simulink model "gm_uz_inverter_3phgm_vnl"  (R2021b)
settings: Solver=FixedStepDiscrete  StartTime=0.0  StopTime=0.6  FixedStep=Auto  RelTol=1e-3
InitFcn:
  | load('C:\Users\valen\Documents\repos\UZ\ultrazohm_sw\ip_cores\uz_inverter_3ph\sschdl\uz_inverter_3ph\stateSpaceParameters.mat');
undefined symbols (not defined in the file or in its folder): g1, g2, g3, g4, g5, g6, i_a, i_b, i_c, pslcontrol, stateSpaceParameters_1, ts
libraries: hdlmdlgenlib x20, simulink x4, hdlssclib x4
settings Model: Creator=LENOVO  LastModifiedBy=valen
settings SolverCC: AlgebraicLoopSolver=TrustRegion
settings DataIOCC: LimitDataPoints=on  SaveOutput=off  SaveTime=off
settings OptimizationCC: BlockReduction=off  ConditionallyExecuteInputs=off  DefaultParameterBehavior=Inlined  InheritOutputTypeSmallerThanSingle=on  LifeSpan=inf
settings DebuggingCC: AlgebraicLoopMsg=error  InheritedTsInSrcMsg=none  SingleTaskRateTransMsg=error  AllowSymbolicDim=off  StrictBusMsg=ErrorOnBusTreatedAsVector  SFUnexpectedBacktrackingDiag=warning  SFNoUnconditionalDefaultTransitionDiag=warning  SFExecutionAtInitializationDiag=none  SFMachineParentedDataDiag=warning  ArithmeticOperatorsInVariantConditions=warning
settings HardwareCC: ProdBitPerPointer=32  ProdBitPerSizeT=32  ProdBitPerPtrDiffT=32  ProdLargestAtomicFloat=None  ProdIntDivRoundTo=Undefined  ProdEndianess=Unspecified  ProdWordSize=32  ProdHWDeviceType=ASIC/FPGA->ASIC/FPGA  ProdEqTarget=off
settings SFSimCC: SimUseLocalCustomCode=off  CustomCodeUndefinedFunction=UseInterfaceOnly
settings RTWCC: RTWUseLocalCustomCode=off
settings CodeAppCC: StateflowObjectComments=on
settings GRTTargetCC: TargetLangStandard=C89/C90 (ANSI)
settings ConfigComp: CovScope=ReferencedModels  CovMetricSettings=dw  CovSaveCumulativeToWorkspaceVar=on  CovSaveSingleToWorkspaceVar=on  CovExternalEMLEnable=off  CovSFcnEnable=off

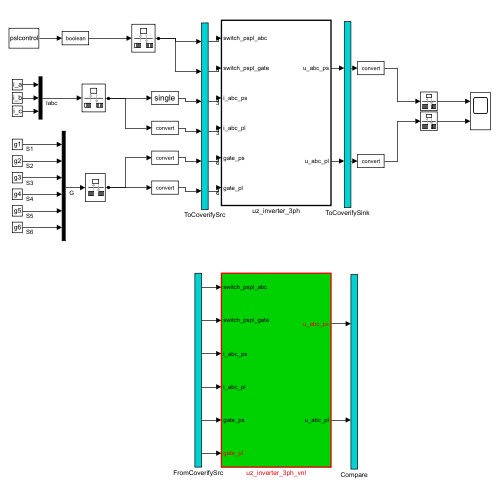
[thumbnail: Simulink's stored preview of the top-level diagram]
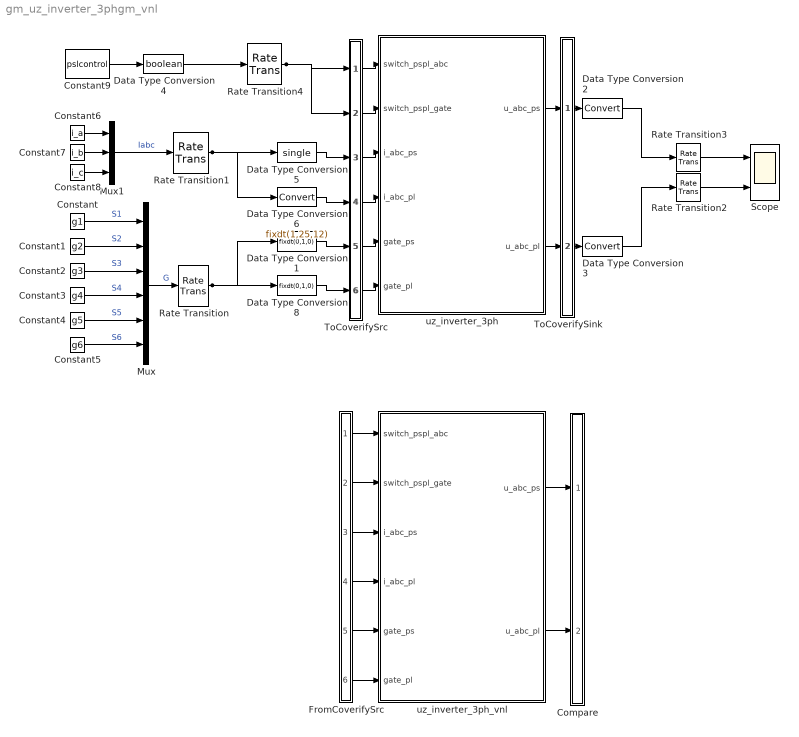
== system gm_uz_inverter_3phgm_vnl ==
  Compare : Subsystem
      mask Display: disp('')
  Constant : Constant  Value=g1  SampleTime=ts
  Constant1 : Constant  Value=g2  SampleTime=ts
  Constant2 : Constant  Value=g3  SampleTime=ts
  Constant3 : Constant  Value=g4  SampleTime=ts
  Constant4 : Constant  Value=g5  SampleTime=ts
  Constant5 : Constant  Value=g6  SampleTime=ts
  Constant6 : Constant  Value=i_a  SampleTime=ts
  Constant7 : Constant  Value=i_b  SampleTime=ts
  Constant8 : Constant  Value=i_c  SampleTime=ts
  Constant9 : Constant  Value=pslcontrol
  Data Type Conversion1 : DataTypeConversion  OutMin=0  OutMax=1  OutDataTypeStr=fixdt(0,1,0)  RndMeth=Nearest
  Data Type Conversion2 : DataTypeConversion
  Data Type Conversion3 : DataTypeConversion
  Data Type Conversion4 : DataTypeConversion  OutDataTypeStr=boolean
  Data Type Conversion5 : DataTypeConversion  OutDataTypeStr=single  RndMeth=Nearest
  Data Type Conversion6 : DataTypeConversion  OutDataTypeStr=fixdt(1,25,12)  RndMeth=Nearest
  Data Type Conversion8 : DataTypeConversion  OutMin=0  OutMax=1  OutDataTypeStr=fixdt(0,1,0)  RndMeth=Nearest
  FromCoverifySrc : Subsystem
      mask Display: disp('')
  Mux : Mux  Inputs=6
  Mux1 : Mux  Inputs=3
  Rate Transition{,1..4} (5 alike) : RateTransition  OutPortSampleTime=ts
  Scope : Scope  NumInputPorts=2
  ToCoverifySink : Subsystem
      mask Display: disp('')
  ToCoverifySrc : Subsystem
      mask Display: disp('')
  uz_inverter_3ph : Subsystem  TreatAsAtomicUnit=on
  uz_inverter_3ph_vnl : Subsystem  TreatAsAtomicUnit=on
  wires:
  Data Type Conversion3/1 -> Rate Transition2/1
  Data Type Conversion2/1 -> Rate Transition3/1
  Rate Transition3/1 -> Scope/1
  Rate Transition2/1 -> Scope/2
  Data Type Conversion4/1 -> Rate Transition4/1
  Constant9/1 -> Data Type Conversion4/1
  Constant2/1 -> Mux/3  "S3"
  Constant4/1 -> Mux/5  "S5"
  Constant5/1 -> Mux/6  "S6"
  Constant3/1 -> Mux/4  "S4"
  Mux1/1 -> Rate Transition1/1  "Iabc"
  Mux/1 -> Rate Transition/1  "G"
  Constant8/1 -> Mux1/3
  Constant6/1 -> Mux1/1
  Constant1/1 -> Mux/2  "S2"
  Constant7/1 -> Mux1/2
  Constant/1 -> Mux/1  "S1"
  Rate Transition1/1 -> Data Type Conversion5/1, Data Type Conversion6/1
  Rate Transition/1 -> Data Type Conversion8/1, Data Type Conversion1/1
  ToCoverifySrc/1(out1) -> uz_inverter_3ph/1(switch_pspl_abc)
  ToCoverifySrc/2(out2) -> uz_inverter_3ph/2(switch_pspl_gate)
  ToCoverifySrc/3(out3) -> uz_inverter_3ph/3(i_abc_ps)
  ToCoverifySrc/4(out4) -> uz_inverter_3ph/4(i_abc_pl)
  ToCoverifySrc/5(out5) -> uz_inverter_3ph/5(gate_ps)
  ToCoverifySrc/6(out6) -> uz_inverter_3ph/6(gate_pl)
  uz_inverter_3ph/1(u_abc_ps) -> ToCoverifySink/1(in1)
  uz_inverter_3ph/2(u_abc_pl) -> ToCoverifySink/2(in2)
  Rate Transition4/1 -> ToCoverifySrc/1(in1), ToCoverifySrc/2(in2)
  Data Type Conversion5/1 -> ToCoverifySrc/3(in3)
  Data Type Conversion6/1 -> ToCoverifySrc/4(in4)
  Data Type Conversion1/1 -> ToCoverifySrc/5(in5)
  Data Type Conversion8/1 -> ToCoverifySrc/6(in6)
  ToCoverifySink/1(out1) -> Data Type Conversion2/1
  ToCoverifySink/2(out2) -> Data Type Conversion3/1
  FromCoverifySrc/1(out1) -> uz_inverter_3ph_vnl/1(switch_pspl_abc)
  FromCoverifySrc/2(out2) -> uz_inverter_3ph_vnl/2(switch_pspl_gate)
  FromCoverifySrc/3(out3) -> uz_inverter_3ph_vnl/3(i_abc_ps)
  FromCoverifySrc/4(out4) -> uz_inverter_3ph_vnl/4(i_abc_pl)
  FromCoverifySrc/5(out5) -> uz_inverter_3ph_vnl/5(gate_ps)
  FromCoverifySrc/6(out6) -> uz_inverter_3ph_vnl/6(gate_pl)
  uz_inverter_3ph_vnl/1(u_abc_ps) -> Compare/1(in1)
  uz_inverter_3ph_vnl/2(u_abc_pl) -> Compare/2(in2)

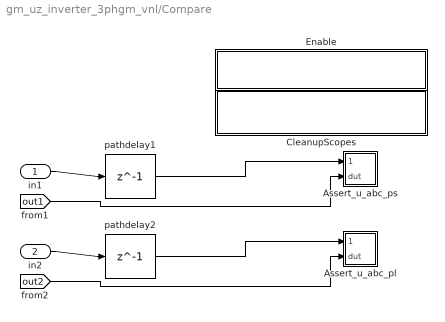
== system gm_uz_inverter_3phgm_vnl/Compare ==
  in1 : Inport
  in2 : Inport  Port=2
  Assert_u_abc_pl : Subsystem
  Assert_u_abc_ps : Subsystem  mask{ToleranceValue=0.001}
  CleanupScopes : Subsystem
      settings: OpenFcn=|
      | blkName = gcb; %self block
      | idx = regexp(blkName, '/CleanupScopes$', 'once');
      | blkParent = blkName(1:idx-1);
      | blks=find_system(blkParent, 'LookUnderMasks', 'all','blocktype', 'Scope');
      | for itr = 1:length(blks)
      | 	 hScopeCfg = get_param(blks{itr},'ScopeConfiguration');
      | 	 hScopeCfg.Visible = ~ hScopeCfg.Visible;
      | end
      | drawnow;
      mask Display: fprintf(message('hdlcoder:cosim:vnl_dblclick').getString());
  Enable : Subsystem
      settings: OpenFcn=|
      | blkName = gcb;
      | idx = regexp(blkName, '/Enable$', 'once');
      | blkParent = blkName(1:idx-1);
      | blks=find_system(blkParent, 'LookUnderMasks', 'all','blocktype', 'Assertion');
      | e = get_param(blks{1}, 'Enabled');
      | if strcmp(e, 'on'), f= 'off';, else, f = 'on';, end
      | for ii=1:length(blks), set_param(blks{ii}, 'Enabled', f);, end
      | set_param(gcb, 'MaskDisplay',['fprintf(message(''hdlcoder:cosim:vnl_dblclick_assertions'',','''',upper(e),'''',').getString())']);
      mask Display: fprintf(message('hdlcoder:cosim:vnl_dblclick_assertions','OFF').getString());
  pathdelay1 : Delay  DelayLength=1
  pathdelay2 : Delay  DelayLength=1
  wires:
  in1/1 -> pathdelay1/1
  pathdelay1/1 -> Assert_u_abc_ps/1(cosim)
  [out1] -> Assert_u_abc_ps/2(dut)
  in2/1 -> pathdelay2/1
  pathdelay2/1 -> Assert_u_abc_pl/1(cosim)
  [out2] -> Assert_u_abc_pl/2(dut)

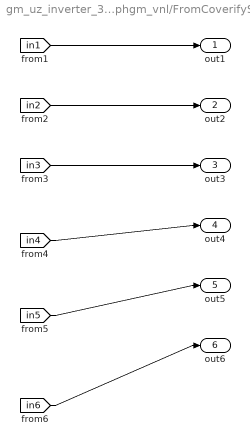
== system gm_uz_inverter_3phgm_vnl/FromCoverifySrc ==
  out1 : Outport
  out2 : Outport  Port=2
  out3 : Outport  Port=3
  out4 : Outport  Port=4
  out5 : Outport  Port=5
  out6 : Outport  Port=6
  wires:
  [in1] -> out1/1
  [in2] -> out2/1
  [in3] -> out3/1
  [in4] -> out4/1
  [in5] -> out5/1
  [in6] -> out6/1

== system gm_uz_inverter_3phgm_vnl/ToCoverifySink ==
  in1 : Inport
  in2 : Inport  Port=2
  out1 : Outport
  out2 : Outport  Port=2
  tag scope: out1=global, out2=global
  wires:
  in1/1 -> out1/1, [out1]
  in2/1 -> out2/1, [out2]

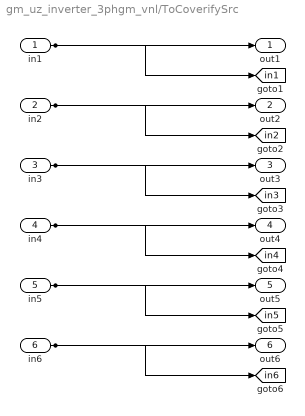
== system gm_uz_inverter_3phgm_vnl/ToCoverifySrc ==
  in1 : Inport
  in2 : Inport  Port=2
  in3 : Inport  Port=3
  in4 : Inport  Port=4
  in5 : Inport  Port=5
  in6 : Inport  Port=6
  out1 : Outport
  out2 : Outport  Port=2
  out3 : Outport  Port=3
  out4 : Outport  Port=4
  out5 : Outport  Port=5
  out6 : Outport  Port=6
  tag scope: in1=global, in2=global, in3=global, in4=global, in5=global, in6=global
  wires:
  in1/1 -> out1/1, [in1]
  in2/1 -> out2/1, [in2]
  in3/1 -> out3/1, [in3]
  in4/1 -> out4/1, [in4]
  in5/1 -> out5/1, [in5]
  in6/1 -> out6/1, [in6]

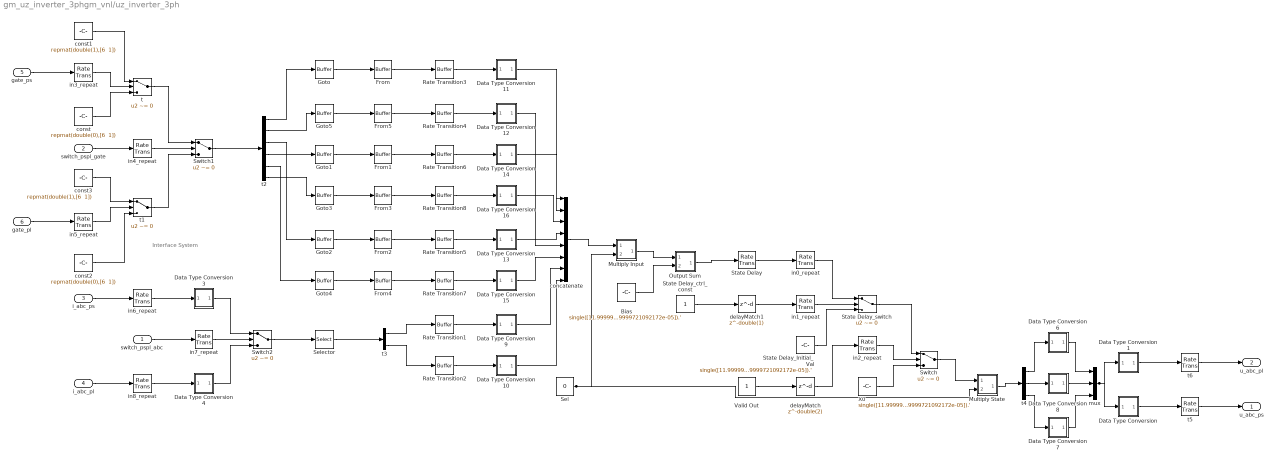
== system gm_uz_inverter_3phgm_vnl/uz_inverter_3ph ==
  note: Interface System
  switch_pspl_abc : Inport  OutDataTypeStr=boolean  PortDimensions=1  SampleTime=5e-07
  switch_pspl_gate : Inport  Port=2  OutDataTypeStr=boolean  PortDimensions=1  SampleTime=5e-07
  i_abc_ps : Inport  Port=3  OutDataTypeStr=single  PortDimensions=[3]  SampleTime=5e-07
  i_abc_pl : Inport  Port=4  OutDataTypeStr=fixdt(1, 25, 12)  PortDimensions=[3]  SampleTime=5e-07
  gate_ps : Inport  Port=5  OutDataTypeStr=fixdt(0, 1, 0)  PortDimensions=[6]  SampleTime=5e-07  LockScale=on
  gate_pl : Inport  Port=6  OutDataTypeStr=fixdt(0, 1, 0)  PortDimensions=[6]  SampleTime=5e-07
  Bias : Constant  Value=single([11.99999713897705 -11.99999713897705 0 -0.0002399999793851748 2.399999721092172e-05 -0.00012 1.2e-05 -2.6399995037285073e-11 0.00026399994385428727 0.00026399994385428727 1.2e-05 2.399999721092172e-05]).'  OutDataTypeStr=single  SampleTime=1e-08
  Data Type Conversion : Subsystem
      mask Display: disp('NFP\nconv');
  Data Type Conversion1 : Subsystem
      mask Display: disp('NFP\nconv');
  Data Type Conversion10 : Subsystem
      mask Display: disp('NFP\nconv');
  Data Type Conversion11 : Subsystem
      mask Display: disp('NFP\nconv');
  Data Type Conversion12 : Subsystem
      mask Display: disp('NFP\nconv');
  Data Type Conversion13 : Subsystem
      mask Display: disp('NFP\nconv');
  Data Type Conversion14 : Subsystem
      mask Display: disp('NFP\nconv');
  Data Type Conversion15 : Subsystem
      mask Display: disp('NFP\nconv');
  Data Type Conversion16 : Subsystem
      mask Display: disp('NFP\nconv');
  Data Type Conversion3 : Subsystem
      mask Display: disp('NFP\nconv');
  Data Type Conversion4 : Subsystem
      mask Display: disp('NFP\nconv');
  Data Type Conversion6 : Subsystem
      mask Display: disp('NFP\nconv');
  Data Type Conversion7 : Subsystem
      mask Display: disp('NFP\nconv');
  Data Type Conversion8 : Subsystem
      mask Display: disp('NFP\nconv');
  Data Type Conversion9 : Subsystem
      mask Display: disp('NFP\nconv');
  From{,1..5} (6 alike) : hdlmdlgenlib/Buffer
      settings: SourceProductBaseCode=SL
  Goto{,1..5} (6 alike) : hdlmdlgenlib/Buffer
      settings: SourceProductBaseCode=SL
  Multiply Input : Subsystem
      mask Display: disp('NFP\nSparseConstMultiply');
  Multiply State : Subsystem
      mask Display: disp('NFP\nSparseConstMultiply');
  Output Sum : Subsystem
      mask Display: disp('NFP\nadd');
  Rate Transition{1..8} (8 alike) : hdlmdlgenlib/Buffer
      settings: SourceProductBaseCode=SL
  Sel : Constant  Value=0  OutDataTypeStr=uint32  SampleTime=1e-08
  Selector : Selector  SampleTime=1e-08  IndexOptions=Index vector (dialog)  Indices=double([1 2])  OutputSizes=double(1)
  State Delay : RateTransition  OutPortSampleTimeOpt=Multiple of input port sample time  OutPortSampleTimeMultiple=50
  State Delay_Initial_Val : Constant  Value=single([11.99999713897705 -11.99999713897705 6.543061643369901e-16 -0.0002399999793851748 2.399999721092172e-05 -0.00012 1.2e-05 -2.6399995037285073e-11 0.00026399994385428727 0.00026399994385428727 1.2e-05 2.399999721092172e-05]).'  OutDataTypeStr=single  SampleTime=1e-08
  State Delay_ctrl_const : Constant  OutDataTypeStr=boolean  SampleTime=5e-07
  State Delay_switch : Switch  Criteria=u2 ~= 0  Threshold=double(0)  OutDataTypeStr=single  SampleTime=1e-08
  Switch : Switch  Criteria=u2 ~= 0  Threshold=double(0)  OutDataTypeStr=single  SampleTime=1e-08
  Switch1 : Switch  Criteria=u2 ~= 0  Threshold=double(0)  OutDataTypeStr=double  SampleTime=1e-08
  Switch2 : Switch  Criteria=u2 ~= 0  Threshold=double(0)  OutDataTypeStr=double  SampleTime=1e-08
  Valid Out : Constant  OutDataTypeStr=boolean  SampleTime=5e-07
  X0 : Constant  Value=single([11.99999713897705 -11.99999713897705 6.543061643369901e-16 -0.0002399999793851748 2.399999721092172e-05 -0.00012 1.2e-05 -2.6399995037285073e-11 0.00026399994385428727 0.00026399994385428727 1.2e-05 2.399999721092172e-05]).'  OutDataTypeStr=single  SampleTime=1e-08
  concatenate : Concatenate  NumInputs=8
  const : Constant  Value="repmat(double(0),[6  1])"  OutDataTypeStr=double  SampleTime=1e-08
  const1 : Constant  Value="repmat(double(1),[6  1])"  OutDataTypeStr=double  SampleTime=1e-08
  const2 : Constant  Value="repmat(double(0),[6  1])"  OutDataTypeStr=double  SampleTime=1e-08
  const3 : Constant  Value="repmat(double(1),[6  1])"  OutDataTypeStr=double  SampleTime=1e-08
  delayMatch : Delay  DelayLength=double(2)  InitialCondition=0  SampleTime=5e-07
  delayMatch1 : Delay  DelayLength=double(1)  InitialCondition=0  SampleTime=5e-07
  in0_repeat : RateTransition  Integrity=off  Deterministic=off  OutPortSampleTimeOpt=Multiple of input port sample time  OutPortSampleTimeMultiple=1/50
  in1_repeat : RateTransition  Integrity=off  Deterministic=off  OutPortSampleTimeOpt=Multiple of input port sample time  OutPortSampleTimeMultiple=1/50
  in2_repeat : RateTransition  Integrity=off  Deterministic=off  OutPortSampleTimeOpt=Multiple of input port sample time  OutPortSampleTimeMultiple=1/50
  in3_repeat : RateTransition  Integrity=off  Deterministic=off  OutPortSampleTimeOpt=Multiple of input port sample time  OutPortSampleTimeMultiple=1/50
  in4_repeat : RateTransition  Integrity=off  Deterministic=off  OutPortSampleTimeOpt=Multiple of input port sample time  OutPortSampleTimeMultiple=1/50
  in5_repeat : RateTransition  Integrity=off  Deterministic=off  OutPortSampleTimeOpt=Multiple of input port sample time  OutPortSampleTimeMultiple=1/50
  in6_repeat : RateTransition  Integrity=off  Deterministic=off  OutPortSampleTimeOpt=Multiple of input port sample time  OutPortSampleTimeMultiple=1/50
  in7_repeat : RateTransition  Integrity=off  Deterministic=off  OutPortSampleTimeOpt=Multiple of input port sample time  OutPortSampleTimeMultiple=1/50
  in8_repeat : RateTransition  Integrity=off  Deterministic=off  OutPortSampleTimeOpt=Multiple of input port sample time  OutPortSampleTimeMultiple=1/50
  mux : Mux  Inputs=3
  t : Switch  Criteria=u2 ~= 0  Threshold=double(0)  OutDataTypeStr=double  SampleTime=1e-08
  t1 : Switch  Criteria=u2 ~= 0  Threshold=double(0)  OutDataTypeStr=double  SampleTime=1e-08
  t2 : Demux  Outputs=6
  t3 : Demux  Outputs=2
  t4 : Demux  Outputs=3
  t5 : RateTransition  OutPortSampleTimeOpt=Multiple of input port sample time  OutPortSampleTimeMultiple=50
  t6 : RateTransition  OutPortSampleTimeOpt=Multiple of input port sample time  OutPortSampleTimeMultiple=50
  u_abc_ps : Outport  SampleTime=5e-07
  u_abc_pl : Outport  Port=2  OutDataTypeStr=fixdt(1,25,12)  SampleTime=5e-07
  wires:
  Data Type Conversion/1(Out1) -> t5/1
  Data Type Conversion6/1(Out1) -> mux/1
  Multiply State/1(Out1) -> t4/1
  Multiply Input/1(Out1) -> Output Sum/1(In1)
  Data Type Conversion9/1(Out1) -> concatenate/7
  Data Type Conversion4/1(Out1) -> Switch2/3
  Data Type Conversion3/1(Out1) -> Switch2/1
  Data Type Conversion10/1(Out1) -> concatenate/8
  Data Type Conversion11/1(Out1) -> concatenate/1
  Data Type Conversion16/1(Out1) -> concatenate/3
  Data Type Conversion15/1(Out1) -> concatenate/6
  Data Type Conversion14/1(Out1) -> concatenate/2
  Data Type Conversion13/1(Out1) -> concatenate/4
  Data Type Conversion12/1(Out1) -> concatenate/5
  Output Sum/1(Out1) -> State Delay/1
  Data Type Conversion7/1(Out1) -> mux/3
  Data Type Conversion8/1(Out1) -> mux/2
  Data Type Conversion1/1(Out1) -> t6/1
  t4/3 -> Data Type Conversion7/1(In1)
  t4/2 -> Data Type Conversion8/1(In1)
  t4/1 -> Data Type Conversion6/1(In1)
  t3/2 -> Rate Transition2/1
  t3/1 -> Rate Transition1/1
  t2/6 -> Goto3/1
  t2/5 -> Goto4/1
  t2/4 -> Goto1/1
  t2/3 -> Goto2/1
  t2/2 -> Goto5/1
  t2/1 -> Goto/1
  const3/1 -> t1/1
  const2/1 -> t1/3
  const1/1 -> t/1
  const/1 -> t/3
  mux/1 -> Data Type Conversion1/1(In1), Data Type Conversion/1(In1)
  Sel/1 -> Multiply Input/2(In2), Multiply State/2(In2)
  concatenate/1 -> Multiply Input/1(In1)
  Rate Transition1/1 -> Data Type Conversion9/1(In1)
  Selector/1 -> t3/1
  Switch2/1 -> Selector/1
  Rate Transition2/1 -> Data Type Conversion10/1(In1)
  Rate Transition3/1 -> Data Type Conversion11/1(In1)
  From/1 -> Rate Transition3/1
  Goto/1 -> From/1
  Switch1/1 -> t2/1
  t1/1 -> Switch1/3
  t/1 -> Switch1/1
  Goto3/1 -> From3/1
  From3/1 -> Rate Transition8/1
  Rate Transition8/1 -> Data Type Conversion16/1(In1)
  Goto4/1 -> From4/1
  From4/1 -> Rate Transition7/1
  Rate Transition7/1 -> Data Type Conversion15/1(In1)
  Goto1/1 -> From1/1
  From1/1 -> Rate Transition6/1
  Rate Transition6/1 -> Data Type Conversion14/1(In1)
  Goto2/1 -> From2/1
  From2/1 -> Rate Transition5/1
  Rate Transition5/1 -> Data Type Conversion13/1(In1)
  Goto5/1 -> From5/1
  From5/1 -> Rate Transition4/1
  Rate Transition4/1 -> Data Type Conversion12/1(In1)
  Bias/1 -> Output Sum/2(In2)
  Switch/1 -> Multiply State/1(In1)
  X0/1 -> Switch/3
  State Delay_switch/1 -> Switch/1
  State Delay_Initial_Val/1 -> State Delay_switch/3
  in8_repeat/1 -> Data Type Conversion4/1(In1)
  in7_repeat/1 -> Switch2/2
  in6_repeat/1 -> Data Type Conversion3/1(In1)
  in5_repeat/1 -> t1/2
  in4_repeat/1 -> Switch1/2
  in3_repeat/1 -> t/2
  in2_repeat/1 -> Switch/2
  in1_repeat/1 -> State Delay_switch/2
  in0_repeat/1 -> State Delay_switch/1
  State Delay_ctrl_const/1 -> delayMatch1/1
  Valid Out/1 -> delayMatch/1
  State Delay/1 -> in0_repeat/1
  t6/1 -> u_abc_pl/1
  t5/1 -> u_abc_ps/1
  delayMatch1/1 -> in1_repeat/1
  delayMatch/1 -> in2_repeat/1
  gate_pl/1 -> in5_repeat/1
  gate_ps/1 -> in3_repeat/1
  i_abc_pl/1 -> in8_repeat/1
  i_abc_ps/1 -> in6_repeat/1
  switch_pspl_gate/1 -> in4_repeat/1
  switch_pspl_abc/1 -> in7_repeat/1

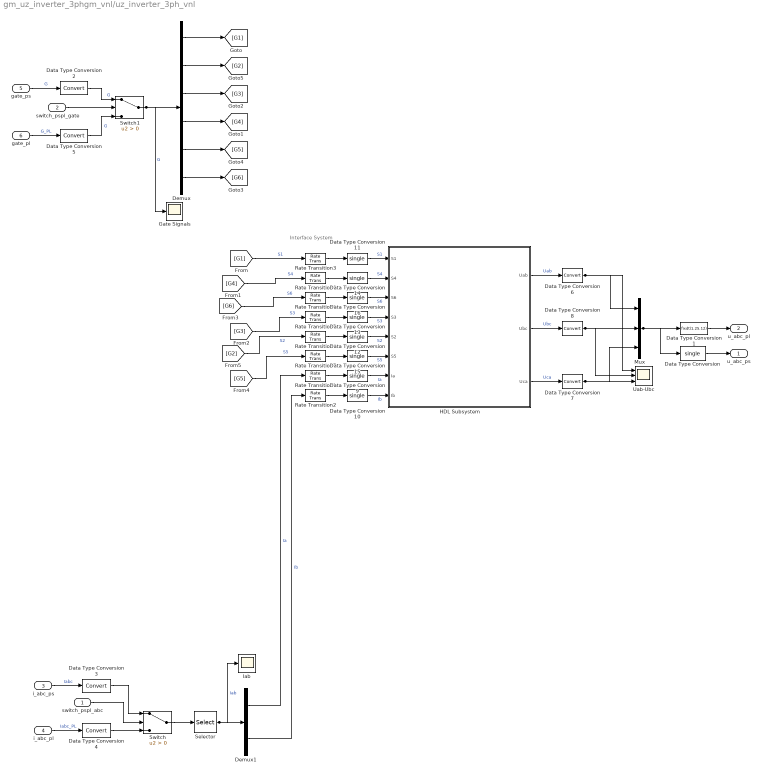
== system gm_uz_inverter_3phgm_vnl/uz_inverter_3ph_vnl ==
  note: Interface System
  switch_pspl_abc : Inport
  switch_pspl_gate : Inport  Port=2
  i_abc_ps : Inport  Port=3  OutDataTypeStr=single
  i_abc_pl : Inport  Port=4  OutDataTypeStr=fixdt(1,25,12)
  gate_ps : Inport  Port=5  OutDataTypeStr=fixdt(0,1,0)  LockScale=on
  gate_pl : Inport  Port=6  OutDataTypeStr=fixdt(0,1,0)
  Data Type Conversion{,9..16} (9 alike) : DataTypeConversion  OutDataTypeStr=single  RndMeth=Nearest
  Data Type Conversion1 : DataTypeConversion  OutDataTypeStr=fixdt(1,25,12)  RndMeth=Nearest
  Data Type Conversion{2..8} (7 alike) : DataTypeConversion  RndMeth=Nearest
  Demux : Demux  Outputs=6
  Demux1 : Demux  Outputs=2
  Gate Signals : Scope
  HDL Subsystem : Subsystem
  Iab : Scope
  Mux : Mux  Inputs=3
  Rate Transition{1..8} (8 alike) : RateTransition  OutPortSampleTime=5e-07
  Selector : Selector  InputPortWidth=3  IndexOptions=Index vector (dialog)  Indices=[1 2]  OutputSizes=1
  Switch : Switch  Criteria=u2 > Threshold
  Switch1 : Switch  Criteria=u2 > Threshold
  Uab-Ubc : Scope  NumInputPorts=3
  u_abc_ps : Outport
  u_abc_pl : Outport  Port=2  OutDataTypeStr=fixdt(1,25,12)
  wires:
  [G1] -> Rate Transition3/1  "S1"
  [G2] -> Rate Transition4/1  "S2"
  [G6] -> Rate Transition8/1  "S6"
  [G5] -> Rate Transition7/1  "S5"
  HDL Subsystem/1(Uab) -> Data Type Conversion6/1  "Uab"
  HDL Subsystem/3(Uca) -> Data Type Conversion7/1  "Uca"
  HDL Subsystem/2(Ubc) -> Data Type Conversion8/1  "Ubc"
  Demux1/1 -> Rate Transition1/1  "Ia"
  [G3] -> Rate Transition5/1  "S3"
  Demux1/2 -> Rate Transition2/1  "Ib"
  [G4] -> Rate Transition6/1  "S4"
  Rate Transition2/1 -> Data Type Conversion10/1
  Rate Transition4/1 -> Data Type Conversion12/1
  Rate Transition1/1 -> Data Type Conversion9/1
  Rate Transition5/1 -> Data Type Conversion13/1
  Rate Transition8/1 -> Data Type Conversion16/1
  Data Type Conversion11/1 -> HDL Subsystem/1(S1)  "S1"
  Data Type Conversion14/1 -> HDL Subsystem/2(S4)  "S4"
  Data Type Conversion16/1 -> HDL Subsystem/3(S6)  "S6"
  Rate Transition3/1 -> Data Type Conversion11/1
  Data Type Conversion15/1 -> HDL Subsystem/6(S5)  "S5"
  Data Type Conversion12/1 -> HDL Subsystem/5(S2)  "S2"
  Data Type Conversion13/1 -> HDL Subsystem/4(S3)  "S3"
  i_abc_ps/1 -> Data Type Conversion3/1  "Iabc"
  Data Type Conversion9/1 -> HDL Subsystem/7(Ia)  "Ia"
  switch_pspl_abc/1 -> Switch/2
  Selector/1 -> Iab/1, Demux1/1  "Iab"
  Rate Transition6/1 -> Data Type Conversion14/1
  Demux/3 -> [G3]
  Data Type Conversion3/1 -> Switch/1
  Demux/1 -> [G1]
  Data Type Conversion4/1 -> Switch/3
  gate_ps/1 -> Data Type Conversion2/1  "G"
  Rate Transition7/1 -> Data Type Conversion15/1
  Data Type Conversion10/1 -> HDL Subsystem/8(Ib)  "Ib"
  switch_pspl_gate/1 -> Switch1/2
  Demux/6 -> [G6]
  gate_pl/1 -> Data Type Conversion5/1  "G_PL"
  Demux/4 -> [G4]
  Data Type Conversion1/1 -> u_abc_pl/1
  Mux/1 -> Data Type Conversion1/1, Data Type Conversion/1
  Data Type Conversion/1 -> u_abc_ps/1
  Data Type Conversion5/1 -> Switch1/3  "G"
  Demux/5 -> [G5]
  Data Type Conversion8/1 -> Uab-Ubc/2, Mux/2
  i_abc_pl/1 -> Data Type Conversion4/1  "Iabc_PL"
  Data Type Conversion7/1 -> Mux/3, Uab-Ubc/3
  Switch/1 -> Selector/1
  Data Type Conversion6/1 -> Uab-Ubc/1, Mux/1
  Switch1/1 -> Gate Signals/1, Demux/1  "G"
  Data Type Conversion2/1 -> Switch1/1  "G"
  Demux/2 -> [G2]

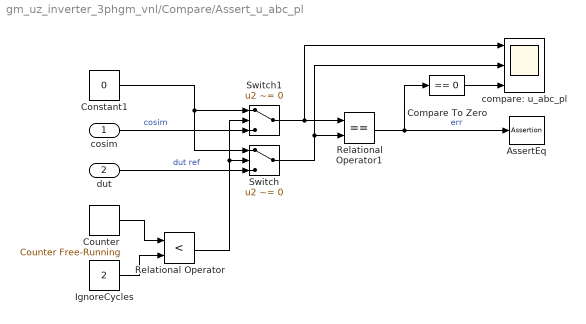
== system gm_uz_inverter_3phgm_vnl/Compare/Assert_u_abc_pl ==
  cosim : Inport
  dut : Inport  Port=2
  AssertEq : Assertion  StopWhenAssertionFail=off
  Compare To Zero : simulink/Logic and Bit Operations/Compare To Zero  relop===  OutDataTypeStr=boolean
  Constant1 : Constant  Value=0  OutDataTypeStr=Inherit: Inherit via back propagation  SampleTime=-1
  Counter : simulink/Sources/Counter Free-Running  NumBits=32  tsamp=-1
  IgnoreCycles : Constant  Value=2  OutDataTypeStr=Inherit: Inherit via back propagation  SampleTime=-1
  Relational Operator : RelationalOperator  Operator=<  OutDataTypeStr=boolean  RndMeth=Nearest
  Relational Operator1 : RelationalOperator  Operator===  OutDataTypeStr=boolean  RndMeth=Nearest
  Switch : Switch  Criteria=u2 ~= 0
  Switch1 : Switch  Criteria=u2 ~= 0
  compare: u_abc_pl : Scope  NumInputPorts=3
  wires:
  Compare To Zero/1 -> compare: u_abc_pl/3
  Relational Operator1/1 -> Compare To Zero/1, AssertEq/1  "err"
  Switch1/1 -> compare: u_abc_pl/1, Relational Operator1/1
  Switch/1 -> compare: u_abc_pl/2, Relational Operator1/2
  Constant1/1 -> Switch/1, Switch1/1
  Relational Operator/1 -> Switch/2, Switch1/2
  cosim/1 -> Switch1/3  "cosim"
  dut/1 -> Switch/3  "dut ref"
  Counter/1 -> Relational Operator/1
  IgnoreCycles/1 -> Relational Operator/2

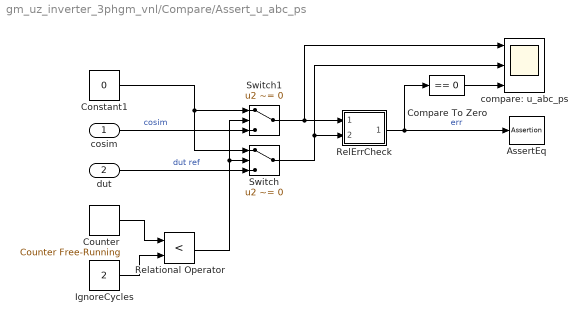
== system gm_uz_inverter_3phgm_vnl/Compare/Assert_u_abc_ps ==
  cosim : Inport
  dut : Inport  Port=2
  AssertEq : Assertion  StopWhenAssertionFail=off
  Compare To Zero : simulink/Logic and Bit Operations/Compare To Zero  relop===  OutDataTypeStr=boolean
  Constant1 : Constant  Value=0  OutDataTypeStr=Inherit: Inherit via back propagation  SampleTime=-1
  Counter : simulink/Sources/Counter Free-Running  NumBits=32  tsamp=-1
  IgnoreCycles : Constant  Value=2  OutDataTypeStr=Inherit: Inherit via back propagation  SampleTime=-1
  RelErrCheck : Subsystem
  Relational Operator : RelationalOperator  Operator=<  OutDataTypeStr=boolean  RndMeth=Nearest
  Switch : Switch  Criteria=u2 ~= 0
  Switch1 : Switch  Criteria=u2 ~= 0
  compare: u_abc_ps : Scope  NumInputPorts=3
  wires:
  IgnoreCycles/1 -> Relational Operator/2
  Counter/1 -> Relational Operator/1
  dut/1 -> Switch/3  "dut ref"
  cosim/1 -> Switch1/3  "cosim"
  Relational Operator/1 -> Switch1/2, Switch/2
  Constant1/1 -> Switch1/1, Switch/1
  Switch/1 -> compare: u_abc_ps/2, RelErrCheck/2(In2)
  Switch1/1 -> compare: u_abc_ps/1, RelErrCheck/1(In1)
  RelErrCheck/1(Out1) -> AssertEq/1, Compare To Zero/1  "err"
  Compare To Zero/1 -> compare: u_abc_ps/3

== system gm_uz_inverter_3phgm_vnl/Compare/CleanupScopes ==

== system gm_uz_inverter_3phgm_vnl/Compare/Enable ==

== system gm_uz_inverter_3phgm_vnl/uz_inverter_3ph/Data Type Conversion ==
  In1 : Inport
  Data Type Conversion : DataTypeConversion  OutDataTypeStr=single  RndMeth=Nearest  SampleTime=1e-08
  Data Type Conversion_pd1 : Delay  DelayLength=3
  Out1 : Outport
  wires:
  Data Type Conversion_pd1/1 -> Out1/1
  Data Type Conversion/1 -> Data Type Conversion_pd1/1
  In1/1 -> Data Type Conversion/1

== system gm_uz_inverter_3phgm_vnl/uz_inverter_3ph/Data Type Conversion1 ==
  In1 : Inport
  Data Type Conversion1 : DataTypeConversion  OutDataTypeStr=fixdt(1, 25, 12)  RndMeth=Nearest  SampleTime=1e-08
  Data Type Conversion1_pd1 : Delay  DelayLength=3
  Out1 : Outport
  wires:
  Data Type Conversion1_pd1/1 -> Out1/1
  Data Type Conversion1/1 -> Data Type Conversion1_pd1/1
  In1/1 -> Data Type Conversion1/1

== system gm_uz_inverter_3phgm_vnl/uz_inverter_3ph/Data Type Conversion10 ==
  In1 : Inport
  Data Type Conversion10 : DataTypeConversion  OutDataTypeStr=single  RndMeth=Nearest  SampleTime=1e-08
  Data Type Conversion10_pd1 : Delay  DelayLength=3
  Out1 : Outport
  wires:
  Data Type Conversion10_pd1/1 -> Out1/1
  Data Type Conversion10/1 -> Data Type Conversion10_pd1/1
  In1/1 -> Data Type Conversion10/1

== system gm_uz_inverter_3phgm_vnl/uz_inverter_3ph/Data Type Conversion11 ==
  In1 : Inport
  Data Type Conversion11 : DataTypeConversion  OutDataTypeStr=single  RndMeth=Nearest  SampleTime=1e-08
  Data Type Conversion11_pd1 : Delay  DelayLength=3
  Out1 : Outport
  wires:
  Data Type Conversion11_pd1/1 -> Out1/1
  Data Type Conversion11/1 -> Data Type Conversion11_pd1/1
  In1/1 -> Data Type Conversion11/1

== system gm_uz_inverter_3phgm_vnl/uz_inverter_3ph/Data Type Conversion12 ==
  In1 : Inport
  Data Type Conversion12 : DataTypeConversion  OutDataTypeStr=single  RndMeth=Nearest  SampleTime=1e-08
  Data Type Conversion12_pd1 : Delay  DelayLength=3
  Out1 : Outport
  wires:
  Data Type Conversion12_pd1/1 -> Out1/1
  Data Type Conversion12/1 -> Data Type Conversion12_pd1/1
  In1/1 -> Data Type Conversion12/1

== system gm_uz_inverter_3phgm_vnl/uz_inverter_3ph/Data Type Conversion13 ==
  In1 : Inport
  Data Type Conversion13 : DataTypeConversion  OutDataTypeStr=single  RndMeth=Nearest  SampleTime=1e-08
  Data Type Conversion13_pd1 : Delay  DelayLength=3
  Out1 : Outport
  wires:
  Data Type Conversion13_pd1/1 -> Out1/1
  Data Type Conversion13/1 -> Data Type Conversion13_pd1/1
  In1/1 -> Data Type Conversion13/1

== system gm_uz_inverter_3phgm_vnl/uz_inverter_3ph/Data Type Conversion14 ==
  In1 : Inport
  Data Type Conversion14 : DataTypeConversion  OutDataTypeStr=single  RndMeth=Nearest  SampleTime=1e-08
  Data Type Conversion14_pd1 : Delay  DelayLength=3
  Out1 : Outport
  wires:
  Data Type Conversion14_pd1/1 -> Out1/1
  Data Type Conversion14/1 -> Data Type Conversion14_pd1/1
  In1/1 -> Data Type Conversion14/1

== system gm_uz_inverter_3phgm_vnl/uz_inverter_3ph/Data Type Conversion15 ==
  In1 : Inport
  Data Type Conversion15 : DataTypeConversion  OutDataTypeStr=single  RndMeth=Nearest  SampleTime=1e-08
  Data Type Conversion15_pd1 : Delay  DelayLength=3
  Out1 : Outport
  wires:
  Data Type Conversion15_pd1/1 -> Out1/1
  Data Type Conversion15/1 -> Data Type Conversion15_pd1/1
  In1/1 -> Data Type Conversion15/1

== system gm_uz_inverter_3phgm_vnl/uz_inverter_3ph/Data Type Conversion16 ==
  In1 : Inport
  Data Type Conversion16 : DataTypeConversion  OutDataTypeStr=single  RndMeth=Nearest  SampleTime=1e-08
  Data Type Conversion16_pd1 : Delay  DelayLength=3
  Out1 : Outport
  wires:
  Data Type Conversion16_pd1/1 -> Out1/1
  Data Type Conversion16/1 -> Data Type Conversion16_pd1/1
  In1/1 -> Data Type Conversion16/1

== system gm_uz_inverter_3phgm_vnl/uz_inverter_3ph/Data Type Conversion3 ==
  In1 : Inport
  Data Type Conversion3 : DataTypeConversion  OutDataTypeStr=double  RndMeth=Nearest  SampleTime=1e-08
  Data Type Conversion3_pd1 : Delay  DelayLength=3
  Out1 : Outport
  wires:
  Data Type Conversion3_pd1/1 -> Out1/1
  Data Type Conversion3/1 -> Data Type Conversion3_pd1/1
  In1/1 -> Data Type Conversion3/1

== system gm_uz_inverter_3phgm_vnl/uz_inverter_3ph/Data Type Conversion4 ==
  In1 : Inport
  Data Type Conversion4 : DataTypeConversion  OutDataTypeStr=double  RndMeth=Nearest  SampleTime=1e-08
  Data Type Conversion4_pd1 : Delay  DelayLength=3
  Out1 : Outport
  wires:
  Data Type Conversion4_pd1/1 -> Out1/1
  Data Type Conversion4/1 -> Data Type Conversion4_pd1/1
  In1/1 -> Data Type Conversion4/1

== system gm_uz_inverter_3phgm_vnl/uz_inverter_3ph/Data Type Conversion6 ==
  In1 : Inport
  Data Type Conversion6 : DataTypeConversion  OutDataTypeStr=double  RndMeth=Nearest  SampleTime=1e-08
  Data Type Conversion6_pd1 : Delay  DelayLength=3
  Out1 : Outport
  wires:
  Data Type Conversion6_pd1/1 -> Out1/1
  Data Type Conversion6/1 -> Data Type Conversion6_pd1/1
  In1/1 -> Data Type Conversion6/1

== system gm_uz_inverter_3phgm_vnl/uz_inverter_3ph/Data Type Conversion7 ==
  In1 : Inport
  Data Type Conversion7 : DataTypeConversion  OutDataTypeStr=double  RndMeth=Nearest  SampleTime=1e-08
  Data Type Conversion7_pd1 : Delay  DelayLength=3
  Out1 : Outport
  wires:
  Data Type Conversion7_pd1/1 -> Out1/1
  Data Type Conversion7/1 -> Data Type Conversion7_pd1/1
  In1/1 -> Data Type Conversion7/1

== system gm_uz_inverter_3phgm_vnl/uz_inverter_3ph/Data Type Conversion8 ==
  In1 : Inport
  Data Type Conversion8 : DataTypeConversion  OutDataTypeStr=double  RndMeth=Nearest  SampleTime=1e-08
  Data Type Conversion8_pd1 : Delay  DelayLength=3
  Out1 : Outport
  wires:
  Data Type Conversion8_pd1/1 -> Out1/1
  Data Type Conversion8/1 -> Data Type Conversion8_pd1/1
  In1/1 -> Data Type Conversion8/1

== system gm_uz_inverter_3phgm_vnl/uz_inverter_3ph/Data Type Conversion9 ==
  In1 : Inport
  Data Type Conversion9 : DataTypeConversion  OutDataTypeStr=single  RndMeth=Nearest  SampleTime=1e-08
  Data Type Conversion9_pd1 : Delay  DelayLength=3
  Out1 : Outport
  wires:
  Data Type Conversion9_pd1/1 -> Out1/1
  Data Type Conversion9/1 -> Data Type Conversion9_pd1/1
  In1/1 -> Data Type Conversion9/1

== system gm_uz_inverter_3phgm_vnl/uz_inverter_3ph/Multiply Input ==
  In1 : Inport
  In2 : Inport  Port=2
  Multiply Input : hdlssclib/NFPSparseConstMultiply  constMatrix="reshape(single([0 0 0 0 0 0 0 0 0 0 0 0 0 0 0 0 0 0 0 0 0 0 0 0 0 0 0 0 0 0 0 0 0 0 0 0 0 0 0 0 0 0 0 0 0 0 0 0 0 0 0 0 0 0 0 0 0 0 0 0 0 0 0 0 0 0 0 0 0 0 0 0 -0.009999997913837433 0 45454.5469 9.999997985232767e-08 -9.999998162868451e-09 0.4545454680919647 -0.04545454680919647 0 0 0.9999997615814209 0.04545454680919647 0 0 -0.009999997913837433 45454.5469 0 0 0.4545454680919647 -0.04545454680919647 9.999997985232767e-08 -0.9999997615814209 0 0.04545454680919647 9.999998162868451e-09]).', [12   8])"
      settings: SourceProductBaseCode=SL
  Multiply Input_pd1 : Delay  DelayLength=12
  Out1 : Outport
  wires:
  Multiply Input_pd1/1 -> Out1/1
  Multiply Input/1 -> Multiply Input_pd1/1
  In2/1 -> Multiply Input/2
  In1/1 -> Multiply Input/1

== system gm_uz_inverter_3phgm_vnl/uz_inverter_3ph/Multiply State ==
  In1 : Inport
  In2 : Inport  Port=2
  Multiply State : hdlssclib/NFPSparseConstMultiply  constMatrix="reshape(single([1 0 -1 0 1 0 0 0 0 0 0 0 0 0 0 0 0 0 0 0 0 0 0 0 0 0 0 0 0 0 0 0 0 0 0 0]).', [3  12])"
      settings: SourceProductBaseCode=SL
  Multiply State_pd1 : Delay  DelayLength=6
  Out1 : Outport
  wires:
  Multiply State_pd1/1 -> Out1/1
  Multiply State/1 -> Multiply State_pd1/1
  In2/1 -> Multiply State/2
  In1/1 -> Multiply State/1

== system gm_uz_inverter_3phgm_vnl/uz_inverter_3ph/Output Sum ==
  In1 : Inport
  In2 : Inport  Port=2
  Output Sum : Sum  OutDataTypeStr=single  SampleTime=1e-08
  Output Sum_pd1 : Delay  DelayLength=6
  Out1 : Outport
  wires:
  Output Sum_pd1/1 -> Out1/1
  Output Sum/1 -> Output Sum_pd1/1
  In2/1 -> Output Sum/2
  In1/1 -> Output Sum/1

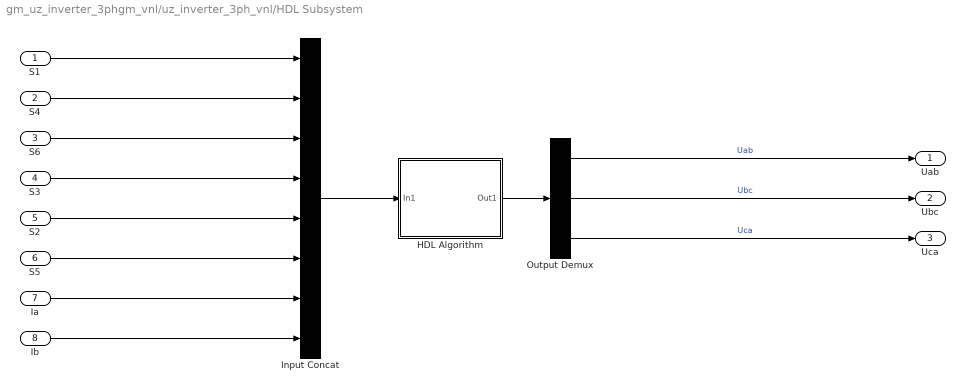
== system gm_uz_inverter_3phgm_vnl/uz_inverter_3ph_vnl/HDL Subsystem ==
  S1 : Inport
  S4 : Inport  Port=2
  S6 : Inport  Port=3
  S3 : Inport  Port=4
  S2 : Inport  Port=5
  S5 : Inport  Port=6
  Ia : Inport  Port=7
  Ib : Inport  Port=8
  HDL Algorithm : Subsystem
  Input Concat : Concatenate  NumInputs=8
  Output Demux : Demux  Outputs=3
  Uab : Outport
  Ubc : Outport  Port=2
  Uca : Outport  Port=3
  wires:
  S1/1 -> Input Concat/1
  Ib/1 -> Input Concat/8
  Output Demux/2 -> Ubc/1  "Ubc"
  S6/1 -> Input Concat/3
  S4/1 -> Input Concat/2
  Ia/1 -> Input Concat/7
  S3/1 -> Input Concat/4
  HDL Algorithm/1(Out1) -> Output Demux/1
  S2/1 -> Input Concat/5
  S5/1 -> Input Concat/6
  Input Concat/1 -> HDL Algorithm/1(In1)
  Output Demux/1 -> Uab/1  "Uab"
  Output Demux/3 -> Uca/1  "Uca"

== system gm_uz_inverter_3phgm_vnl/Compare/Assert_u_abc_ps/RelErrCheck ==
  In1 : Inport
  In2 : Inport  Port=2
  "RelativeErrorCheck " : MATLAB Function  TreatAsAtomicUnit=on
  Out1 : Outport  VectorParamsAs1DForOutWhenUnconnected=off
  wires:
  "RelativeErrorCheck "/1(y) -> Out1/1
  In1/1 -> "RelativeErrorCheck "/1(P)
  In2/1 -> "RelativeErrorCheck "/2(R)

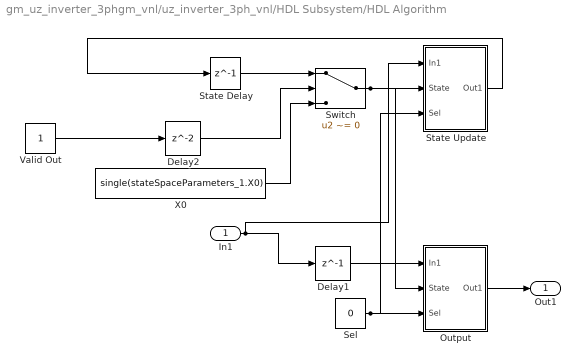
== system gm_uz_inverter_3phgm_vnl/uz_inverter_3ph_vnl/HDL Subsystem/HDL Algorithm ==
  In1 : Inport
  Delay1 : Delay  DelayLength=1
  Delay2 : Delay
  Output : Subsystem
  Sel : Constant  Value=0  OutDataTypeStr=uint32  SampleTime=5e-07
  State Delay : Delay  DelayLength=1  InitialCondition=single(stateSpaceParameters_1.X0)
  State Update : Subsystem
  Switch : Switch  Criteria=u2 ~= 0
  Valid Out : Constant  OutDataTypeStr=boolean  SampleTime=5e-07
  X0 : Constant  Value=single(stateSpaceParameters_1.X0)  SampleTime=5e-07
  Out1 : Outport  VectorParamsAs1DForOutWhenUnconnected=off
  wires:
  Sel/1 -> Output/3(Sel), State Update/3(Sel)
  In1/1 -> Delay1/1, State Update/1(In1)
  Delay1/1 -> Output/1(In1)
  State Update/1(Out1) -> State Delay/1
  State Delay/1 -> Switch/1
  Switch/1 -> Output/2(State), State Update/2(State)
  Output/1(Out1) -> Out1/1
  Delay2/1 -> Switch/2
  Valid Out/1 -> Delay2/1
  X0/1 -> Switch/3

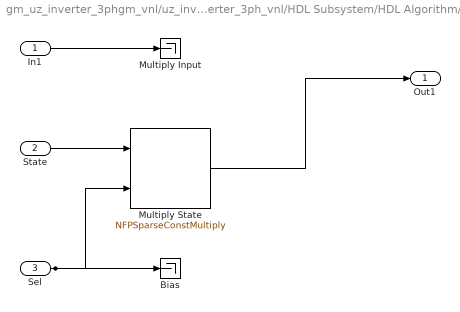
== system gm_uz_inverter_3phgm_vnl/uz_inverter_3ph_vnl/HDL Subsystem/HDL Algorithm/Output ==
  In1 : Inport
  State : Inport  Port=2
  Sel : Inport  Port=3
  Bias : Terminator
  Multiply Input : Terminator
  Multiply State : hdlssclib/NFPSparseConstMultiply  constMatrix=single(stateSpaceParameters_1.Cd)
      settings: SourceProductBaseCode=SL
  Out1 : Outport  VectorParamsAs1DForOutWhenUnconnected=off
  wires:
  Multiply State/1 -> Out1/1
  Sel/1 -> Multiply State/2, Bias/1
  In1/1 -> Multiply Input/1
  State/1 -> Multiply State/1

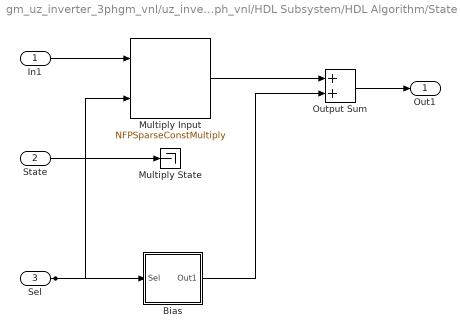
== system gm_uz_inverter_3phgm_vnl/uz_inverter_3ph_vnl/HDL Subsystem/HDL Algorithm/State Update ==
  In1 : Inport
  State : Inport  Port=2
  Sel : Inport  Port=3
  Bias : Subsystem
  Multiply Input : hdlssclib/NFPSparseConstMultiply  constMatrix=single(stateSpaceParameters_1.Bd)
      settings: SourceProductBaseCode=SL
  Multiply State : Terminator
  Output Sum : Sum
  Out1 : Outport  OutDataTypeStr=single  VectorParamsAs1DForOutWhenUnconnected=off
  wires:
  Bias/1(Out1) -> Output Sum/2
  Multiply Input/1 -> Output Sum/1
  Output Sum/1 -> Out1/1
  Sel/1 -> Multiply Input/2, Bias/1(Sel)
  In1/1 -> Multiply Input/1
  State/1 -> Multiply State/1

== system gm_uz_inverter_3phgm_vnl/uz_inverter_3ph_vnl/HDL Subsystem/HDL Algorithm/State Update/Bias ==
  Sel : Inport
  Bias : Constant  Value=single(stateSpaceParameters_1.F0d)  SampleTime=5e-07
  Terminator : Terminator
  Out1 : Outport  VectorParamsAs1DForOutWhenUnconnected=off
  wires:
  Bias/1 -> Out1/1
  Sel/1 -> Terminator/1

== matlab function gm_uz_inverter_3phgm_vnl/Compare/Assert_u_abc_ps/RelErrCheck/RelativeErrorCheck  ==
  data: P input; y output; R input; ToleranceValue parameter double
% Check if the relative error of R with respect to P is below
% ToleranceValue
% P, R are floating-point
function y = relErrCheck(P,R, ToleranceValue)
    tol = ToleranceValue;
    sz = numel(P);
    assert(sz == numel(R), 'Inputs P and R have different sizes.');
    y = false(1, sz);

    for ii=1:sz
        if (isnan(P(ii)) || isnan(R(ii)))
            if (isnan(P(ii)) && isnan(R(ii)))
                y(ii) = true;
            end
        elseif (isinf(P(ii)) || isinf(R(ii)))
            y(ii) = (P(ii) == R(ii));
        elseif (P(ii) == 0)
            y(ii) = (R(ii) == 0);
        else
            absdiff = abs(P(ii) - R(ii));
            relerr = absdiff/abs(P(ii));
            y(ii) = (relerr <= tol);
        end
    end
end
